simulink model "fahrenheitConverter_JamesWilkinson"  (R2025a)
settings: Solver=VariableStepAuto  StartTime=0.0  StopTime=10.0  RelTol=1e-3
settings Model: Creator=james  LastModifiedBy=james

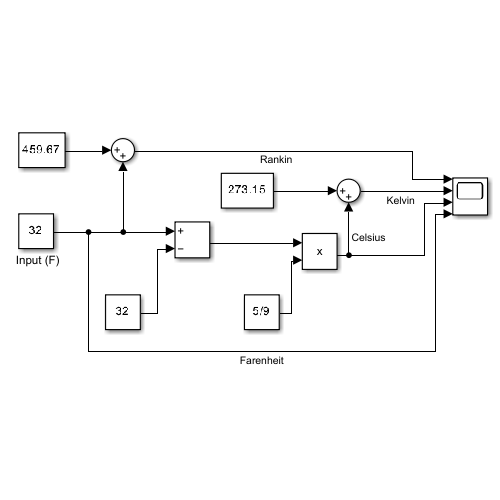
[thumbnail: Simulink's stored preview of the top-level diagram]
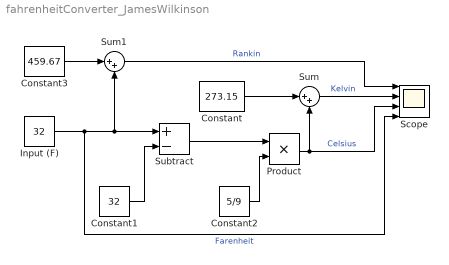
== system fahrenheitConverter_JamesWilkinson ==
  " Input (F)" : Constant  Value=32
  Constant : Constant  Value=273.15
  Constant1 : Constant  Value=32
  Constant2 : Constant  Value=5/9
  Constant3 : Constant  Value=459.67
  Product : Product
  Scope : Scope  NumInputPorts=4
      settings: ActiveDisplayYMinimum=-61.458749999999988  ActiveDisplayYMaximum=553.12875  YLabel=Temp
  Subtract : Sum  Inputs=+-
  Sum : Sum  Inputs=|++
  Sum1 : Sum  Inputs=|++
  wires:
  " Input (F)"/1 -> Sum1/2, Subtract/1, Scope/4  "Farenheit"
  Constant1/1 -> Subtract/2
  Subtract/1 -> Product/1
  Constant2/1 -> Product/2
  Product/1 -> Sum/2, Scope/3  "Celsius"
  Constant/1 -> Sum/1
  Sum/1 -> Scope/2  "Kelvin"
  Sum1/1 -> Scope/1  "Rankin"
  Constant3/1 -> Sum1/1
